simulink model "roket3"  (R2020b)
settings: Solver=VariableStepAuto  StartTime=0.0  StopTime=500  RelTol=1e-3
values from neighbouring files (symbols this model uses):
  Cd = 0.64    [flightdata.m]
  Cm = -0.045    [flightdata.m]
  Cz = 0.08    [flightdata.m]
  d = 0.12    [flightdata.m]
  itki = [2070 2548 2650 2625 2620 2600 2560 2500 2400 2300 2075 1770 1300 700 400]    [flightdata.m]
  Iyy = 78.144    [flightdata.m]
  m = 23.51    [3DOF_Analysis_M2020Cesaroni_Motor_.m]    (also in flightdata.m)
  rho = 1.225    [flightdata.m]
  s = pi*d^2/4    (= 0.0113097335529)    [flightdata.m]
  zaman = [0.023 0.1 0.15 0.2 0.5 1.0 1.5 1.8 2.2 2.5 2.95 3.1 3.3 3.6 3.9]    [flightdata.m]
undefined symbols (not defined in the file or in its folder): magnitude
libraries: simulink x2, sharedtransform x1
settings Model: Creator=ahmet  LastModifiedBy=ahmet

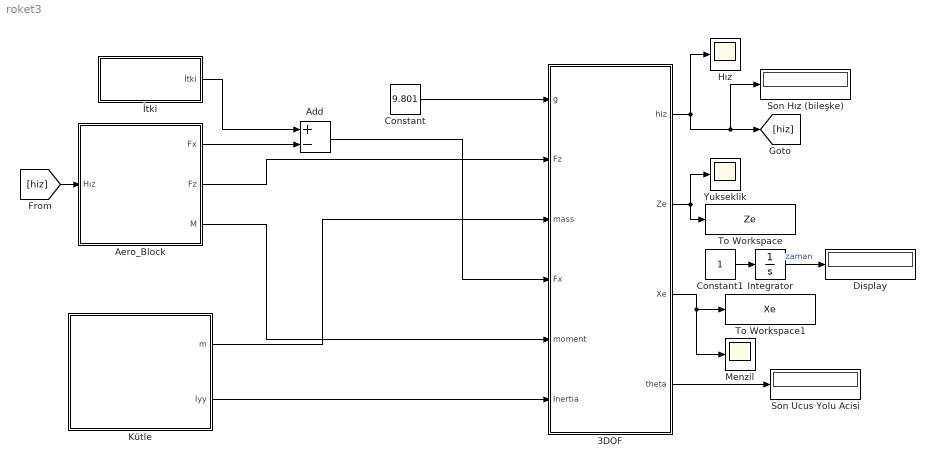
== system roket3 ==
  3DOF : Subsystem
  Add : Sum  Inputs=+-
  Aero_Block : Subsystem
  Constant : Constant  Value=9.801
  Constant1 : Constant
  Display : Display
  Hız : Scope
  Integrator : Integrator
  Kütle : Subsystem
  Menzil : Scope
  Son Hız (bileşke) : Display
  Son Ucus Yolu Acisi : Display
  To Workspace : ToWorkspace  VariableName=Ze  SampleTime=-1
  To Workspace1 : ToWorkspace  VariableName=Xe  SampleTime=-1
  Yukseklik : Scope
  İtki : Subsystem
  wires:
  Constant/1 -> 3DOF/1(g)
  İtki/1(İtki) -> Add/1
  Aero_Block/1(Fx) -> Add/2
  Add/1 -> 3DOF/4(Fx)
  Aero_Block/2(Fz) -> 3DOF/2(Fz)
  Aero_Block/3(M) -> 3DOF/5(moment)
  Kütle/1(m) -> 3DOF/3(mass)
  Kütle/2(Iyy) -> 3DOF/6(Inertia)
  3DOF/1(hiz) -> [hiz], Son Hız (bileşke)/1, Hız/1
  [hiz] -> Aero_Block/1(Hız)
  3DOF/2(Ze) -> To Workspace/1, Yukseklik/1
  3DOF/3(Xe) -> Menzil/1, To Workspace1/1
  Constant1/1 -> Integrator/1
  Integrator/1 -> Display/1  "zaman"
  3DOF/4(theta) -> Son Ucus Yolu Acisi/1

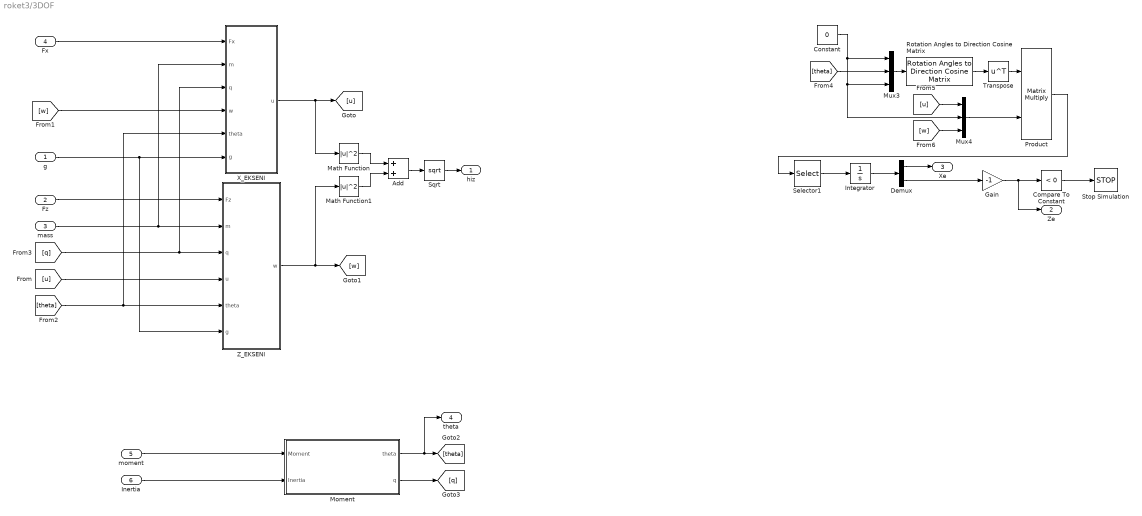
== system roket3/3DOF ==
  g : Inport
  Fz : Inport  Port=2
  mass : Inport  Port=3
  Fx : Inport  Port=4
  moment : Inport  Port=5
  Inertia : Inport  Port=6
  Add : Sum
  Compare To Constant : simulink/Logic and Bit Operations/Compare To Constant  relop=<  const=0  OutDataTypeStr=boolean
  Constant : Constant  Value=0
  Demux : Demux  Outputs=2
  Gain : Gain  Gain=-1
  Integrator : Integrator
  Math Function : Math  Operator=magnitude^2  SaturateOnIntegerOverflow=on
  Math Function1 : Math  Operator=magnitude^2  SaturateOnIntegerOverflow=on
  Moment : Subsystem
  Mux3 : Mux  Inputs=3
  Mux4 : Mux  Inputs=3
  Product : Product  Multiplication=Matrix(*)  SaturateOnIntegerOverflow=on  OutDataTypeStr=Inherit: Same as first input
  Rotation Angles to Direction Cosine Matrix : sharedtransform/Rotation Angles to Direction Cosine Matrix  rotationOrder=ZYX  aMode=aMode
      settings: SourceProductBaseCode=AE,PW,MT,UV,VE,VP
  Selector1 : Selector  InputPortWidth=3  IndexOptions=Index vector (dialog)  Indices=[1 3]  OutputSizes=1
  Sqrt : Sqrt  SaturateOnIntegerOverflow=on
  Stop Simulation : Stop
  Transpose : Math  Operator=transpose  SignedPower=on  SaturateOnIntegerOverflow=on
  X_EKSENI : Subsystem
  Z_EKSENI : Subsystem
  hiz : Outport
  Ze : Outport  Port=2
  Xe : Outport  Port=3
  theta : Outport  Port=4
  wires:
  [theta] -> X_EKSENI/5(theta), Z_EKSENI/5(theta)
  [u] -> Z_EKSENI/4(u)
  [q] -> X_EKSENI/3(q), Z_EKSENI/3(q)
  Fz/1 -> Z_EKSENI/1(Fz)
  mass/1 -> X_EKSENI/2(m), Z_EKSENI/2(m)
  [w] -> X_EKSENI/4(w)
  X_EKSENI/1(u) -> [u], Math Function/1
  g/1 -> Z_EKSENI/6(g), X_EKSENI/6(g)
  Fx/1 -> X_EKSENI/1(Fx)
  Z_EKSENI/1(w) -> [w], Math Function1/1
  Moment/1(theta) -> [theta], theta/1
  moment/1 -> Moment/1(Moment)
  Inertia/1 -> Moment/2(Inertia)
  Moment/2(q) -> [q]
  Math Function/1 -> Add/1
  Math Function1/1 -> Add/2
  Add/1 -> Sqrt/1
  Sqrt/1 -> hiz/1
  [w] -> Mux4/3
  [theta] -> Mux3/2
  Transpose/1 -> Product/1
  Mux4/1 -> Product/2
  Rotation Angles to Direction Cosine Matrix/1 -> Transpose/1
  Constant/1 -> Mux3/1, Mux4/2, Mux3/3
  Product/1 -> Selector1/1
  [u] -> Mux4/1
  Mux3/1 -> Rotation Angles to Direction Cosine Matrix/1
  Selector1/1 -> Integrator/1
  Integrator/1 -> Demux/1
  Demux/2 -> Gain/1
  Gain/1 -> Ze/1, Compare To Constant/1
  Compare To Constant/1 -> Stop Simulation/1
  Demux/1 -> Xe/1

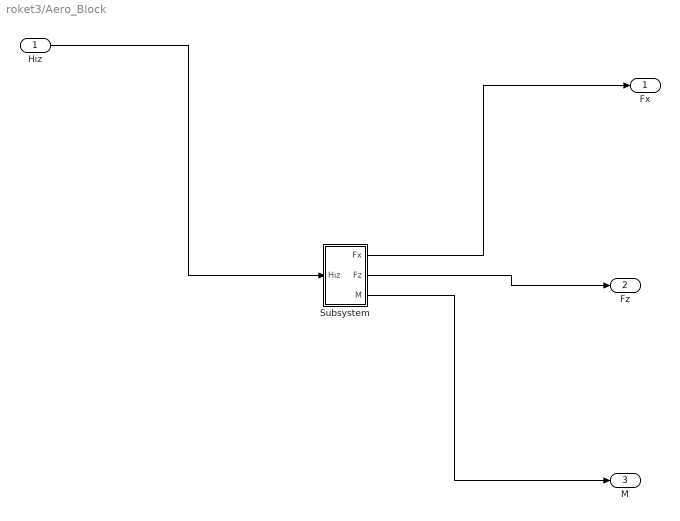
== system roket3/Aero_Block ==
  Hız : Inport
  Subsystem : Subsystem
  Fx : Outport
  Fz : Outport  Port=2
  M : Outport  Port=3
  wires:
  Hız/1 -> Subsystem/1(Hız)
  Subsystem/1(Fx) -> Fx/1
  Subsystem/2(Fz) -> Fz/1
  Subsystem/3(M) -> M/1

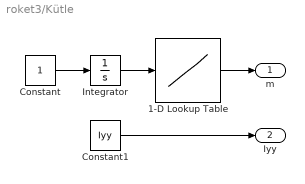
== system roket3/Kütle ==
  1-D Lookup Table : Lookup_n-D  NumberOfTableDimensions=1  BreakpointsForDimension1=[1:1001]  Table=m  InternalRulePriority=Speed  RndMeth=Simplest  InputSameDT=on
  Constant : Constant
  Constant1 : Constant  Value=Iyy
  Integrator : Integrator
  m : Outport
  Iyy : Outport  Port=2
  wires:
  Constant1/1 -> Iyy/1
  1-D Lookup Table/1 -> m/1
  Integrator/1 -> 1-D Lookup Table/1
  Constant/1 -> Integrator/1

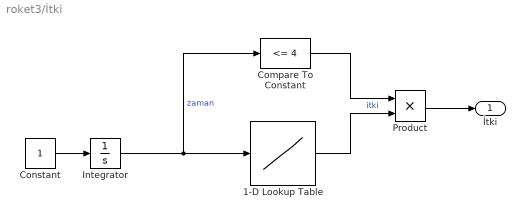
== system roket3/İtki ==
  1-D Lookup Table : Lookup_n-D  NumberOfTableDimensions=1  BreakpointsForDimension1=zaman  Table=itki  InternalRulePriority=Speed  RndMeth=Simplest  InputSameDT=on
  Compare To Constant : simulink/Logic and Bit Operations/Compare To Constant  relop=<=  const=4  OutDataTypeStr=boolean
  Constant : Constant
  Integrator : Integrator
  Product : Product
  İtki : Outport
  wires:
  Constant/1 -> Integrator/1
  1-D Lookup Table/1 -> Product/2  "itki"
  Integrator/1 -> Compare To Constant/1, 1-D Lookup Table/1  "zaman"
  Compare To Constant/1 -> Product/1
  Product/1 -> İtki/1

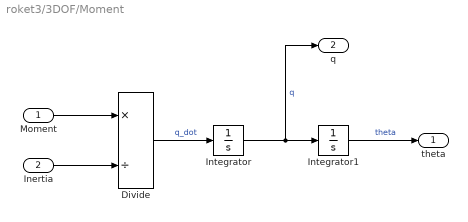
== system roket3/3DOF/Moment ==
  Moment : Inport
  Inertia : Inport  Port=2
  Divide : Product  Inputs=*/
  Integrator : Integrator
  Integrator1 : Integrator  InitialCondition=70*pi/180
  theta : Outport
  q : Outport  Port=2
  wires:
  Integrator/1 -> q/1, Integrator1/1  "q"
  Divide/1 -> Integrator/1  "q_dot"
  Integrator1/1 -> theta/1  "theta"
  Inertia/1 -> Divide/2
  Moment/1 -> Divide/1

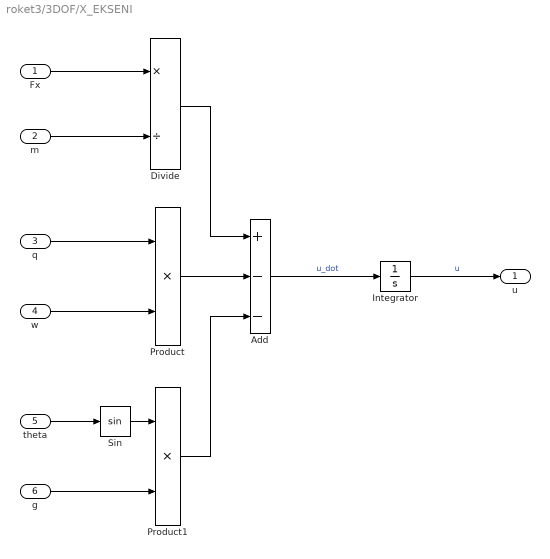
== system roket3/3DOF/X_EKSENI ==
  Fx : Inport
  m : Inport  Port=2
  q : Inport  Port=3
  w : Inport  Port=4
  theta : Inport  Port=5
  g : Inport  Port=6
  Add : Sum  Inputs=+--
  Divide : Product  Inputs=*/
  Integrator : Integrator
  Product : Product
  Product1 : Product
  Sin : Trigonometry
  u : Outport
  wires:
  Divide/1 -> Add/1
  m/1 -> Divide/2
  Fx/1 -> Divide/1
  Sin/1 -> Product1/1
  q/1 -> Product/1
  Add/1 -> Integrator/1  "u_dot"
  Product1/1 -> Add/3
  g/1 -> Product1/2
  Product/1 -> Add/2
  w/1 -> Product/2
  Integrator/1 -> u/1  "u"
  theta/1 -> Sin/1

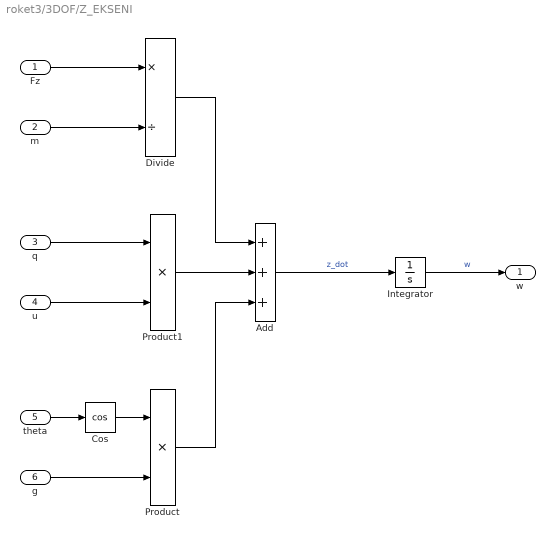
== system roket3/3DOF/Z_EKSENI ==
  Fz : Inport
  m : Inport  Port=2
  q : Inport  Port=3
  u : Inport  Port=4
  theta : Inport  Port=5
  g : Inport  Port=6
  Add : Sum  Inputs=+++
  Cos : Trigonometry  Operator=cos
  Divide : Product  Inputs=*/
  Integrator : Integrator
  Product : Product
  Product1 : Product
  w : Outport
  wires:
  Product/1 -> Add/3
  g/1 -> Product/2
  theta/1 -> Cos/1
  u/1 -> Product1/2
  q/1 -> Product1/1
  m/1 -> Divide/2
  Divide/1 -> Add/1
  Product1/1 -> Add/2
  Fz/1 -> Divide/1
  Integrator/1 -> w/1  "w"
  Add/1 -> Integrator/1  "z_dot"
  Cos/1 -> Product/1

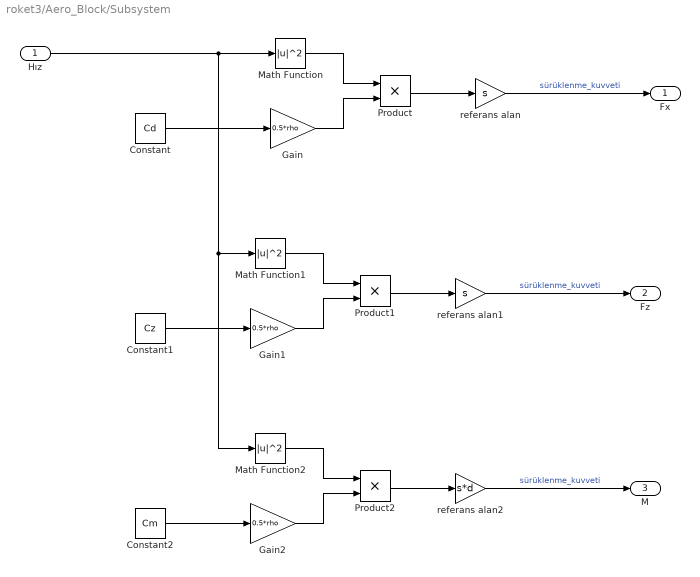
== system roket3/Aero_Block/Subsystem ==
  Hız : Inport
  Constant : Constant  Value=Cd
  Constant1 : Constant  Value=Cz
  Constant2 : Constant  Value=Cm
  Gain : Gain  Gain=0.5*rho
  Gain1 : Gain  Gain=0.5*rho
  Gain2 : Gain  Gain=0.5*rho
  Math Function : Math  Operator=magnitude^2  SaturateOnIntegerOverflow=on
  Math Function1 : Math  Operator=magnitude^2  SaturateOnIntegerOverflow=on
  Math Function2 : Math  Operator=magnitude^2  SaturateOnIntegerOverflow=on
  Product : Product
  Product1 : Product
  Product2 : Product
  referans alan : Gain  Gain=s
  referans alan1 : Gain  Gain=s
  referans alan2 : Gain  Gain=s*d
  Fx : Outport
  Fz : Outport  Port=2
  M : Outport  Port=3
  wires:
  Product1/1 -> referans alan1/1
  Math Function1/1 -> Product1/1
  Gain/1 -> Product/2
  Constant2/1 -> Gain2/1
  Constant1/1 -> Gain1/1
  Hız/1 -> Math Function2/1, Math Function1/1, Math Function/1
  Math Function/1 -> Product/1
  referans alan1/1 -> Fz/1  "sürüklenme_kuvveti"
  Gain1/1 -> Product1/2
  Constant/1 -> Gain/1
  referans alan/1 -> Fx/1  "sürüklenme_kuvveti"
  Product2/1 -> referans alan2/1
  Gain2/1 -> Product2/2
  referans alan2/1 -> M/1  "sürüklenme_kuvveti"
  Math Function2/1 -> Product2/1
  Product/1 -> referans alan/1
